simulink model "myMPC"  (R2020b)
settings: Solver=VariableStepAuto  StartTime=0.0  StopTime=7  RelTol=1e-3
values from neighbouring files (symbols this model uses):
  c = [1 0 -0.083]    [versionLivre.m]
  p_ref_all = test2.Data    [versionLivre.m]
undefined symbols (not defined in the file or in its folder): f, K
libraries: SignalEditorBlockLib x1
settings Model: Creator=wangw  LastModifiedBy=wangw

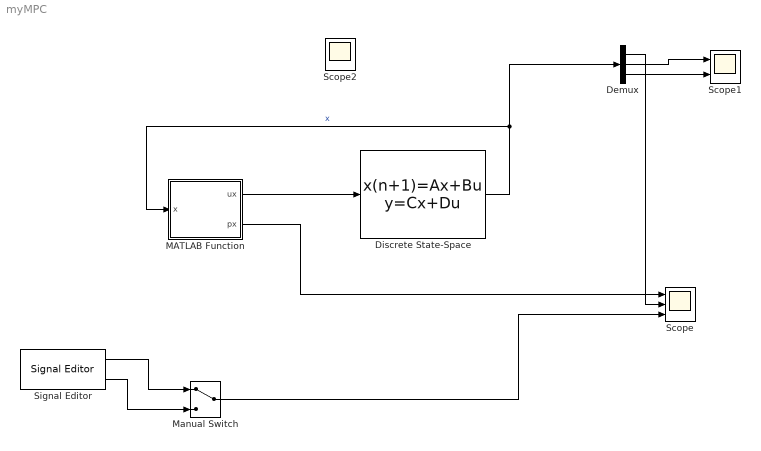
== system myMPC ==
  Demux : Demux  Outputs=3
  Discrete State-Space : DiscreteStateSpace  A=[1, 0.005, 1.25e-05; 0, 1, 0.005; 0, 0, 1]  B=[2.08333e-08; 1.25e-05; 0.005]  C=[1 0 0; 0 1 0; 0 0 1]  D=[0; 0; 0]  SampleTime=0.005
  MATLAB Function : MATLAB Function  TreatAsAtomicUnit=on
  Manual Switch : ManualSwitch
  Scope : Scope  NumInputPorts=3
  Scope1 : Scope  NumInputPorts=2
  Scope2 : Scope
  Signal Editor : SignalEditorBlockLib/Signal Editor  FileName=signalCarre.mat  ActiveScenario=Scenario  ActiveSignal=Signal  IsBus=off  OutputBusObjectStr=Bus: BusObject  SampleTime=0.005  Interpolate=off  ZeroCross=off  OutputAfterFinalValue=Holding final value  Unit=inherit  PreserveSignalName=on
  wires:
  MATLAB Function/1(ux) -> Discrete State-Space/1
  Discrete State-Space/1 -> Demux/1, MATLAB Function/1(x)  "x"
  MATLAB Function/2(px) -> Scope/1
  Demux/1 -> Scope/2
  Demux/2 -> Scope1/1
  Demux/3 -> Scope1/2
  Manual Switch/1 -> Scope/3
  Signal Editor/1 -> Manual Switch/1
  Signal Editor/2 -> Manual Switch/2

== matlab function myMPC/MATLAB Function ==
  data: ux output; x input; p_ref_all parameter size=2001; K parameter size=1 3; f parameter size=160; px output; c parameter
function [ux,px]= My_MPC(x, p_ref_all, K, f, c)
NL = 320;
Nl = 160
persistent k;
    if isempty(k)
            k = 1;
            x = [0;0;0];
    end
p_ref = p_ref_all(k : k+Nl-1);

ux = -K*x + transpose(f)*p_ref;
px = c*x;
k = k+1;
